simulink model "six_phase_half_wave_rectifier"  (R2022a)
settings: Solver=VariableStepAuto  StartTime=0.0  StopTime=0.04  FixedStep=1e-8  RelTol=1e-3
libraries: spsVoltageMeasurementLib x8, spsDetailedThyristorLib x6, spsACVoltageSourceLib x6, spsSeriesRLCBranchLib x1, spsCurrentMeasurementLib x1, spsGroundLib x1, spspowerguiLib x1
settings Model: Creator=alireza  LastModifiedBy=P.O.M.G
settings SolverCC: AlgebraicLoopSolver=TrustRegion
settings DataIOCC: ReturnWorkspaceOutputs=off
settings OptimizationCC: LifeSpan=inf
settings DebuggingCC: UnconnectedInputMsg=warning  UnconnectedOutputMsg=warning  UnconnectedLineMsg=warning  SFExecutionAtInitializationDiag=none  SFMachineParentedDataDiag=warning  ArithmeticOperatorsInVariantConditions=warning
settings SFSimCC: CustomCodeUndefinedFunction=UseInterfaceOnly
settings CodeAppCC: StateflowObjectComments=on

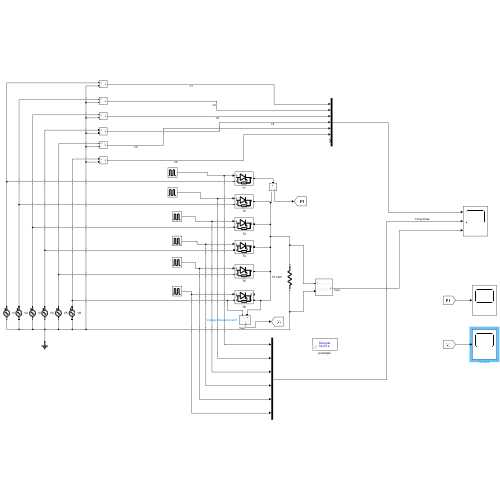
[thumbnail: Simulink's stored preview of the top-level diagram]
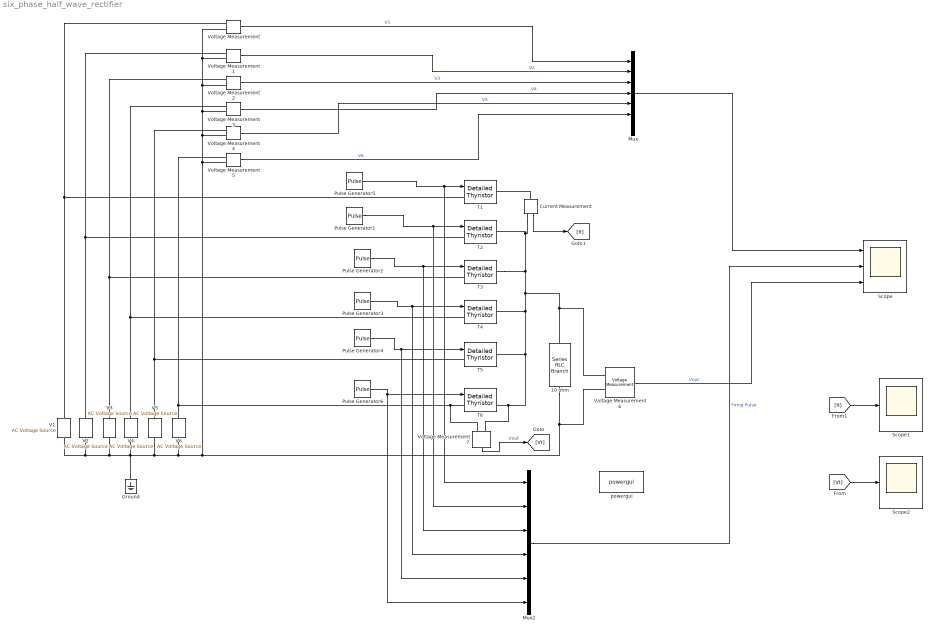
== system six_phase_half_wave_rectifier ==
  10 ohm : spsSeriesRLCBranchLib/Series RLC Branch  LConnTagsString=__new0  RConnTagsString=__new0  BranchType=R  Resistance=10  Inductance=1e-3  SetiL0=off  InitialCurrent=0  Capacitance=1e-6  Setx0=off  InitialVoltage=0  Measurements=None
  Current Measurement : spsCurrentMeasurementLib/Current Measurement  PhasorSimulation=off  OutputType=Complex  PSBequivalent=0
  Ground : spsGroundLib/Ground  LConnTagsString=a
  Mux : Mux  Inputs=7
  Mux2 : Mux  Inputs=6
  Pulse Generator1 : DiscretePulseGenerator  PulseType=Time based  Period=0.02  PulseWidth=5  PhaseDelay=0.02
  Pulse Generator2 : DiscretePulseGenerator  PulseType=Time based  Period=0.02  PulseWidth=5  PhaseDelay=0.01667
  Pulse Generator3 : DiscretePulseGenerator  PulseType=Time based  Period=0.02  PulseWidth=5  PhaseDelay=0.01333
  Pulse Generator4 : DiscretePulseGenerator  PulseType=Time based  Period=0.02  PulseWidth=5  PhaseDelay=0.01
  Pulse Generator5 : DiscretePulseGenerator  PulseType=Time based  Period=0.02  PulseWidth=5  PhaseDelay=0.00333
  Pulse Generator6 : DiscretePulseGenerator  PulseType=Time based  Period=0.02  PulseWidth=5  PhaseDelay=0.00667
  Scope : Scope  NumInputPorts=3
  Scope1 : Scope
  Scope2 : Scope
  T{1..5} (5 alike) : spsDetailedThyristorLib/Detailed Thyristor  Ron=0.001  Lon=1e-3  Vf=0.8  IL=0.1  Tq=100e-6  IC=0  Rs=500  Cs=250e-9  Measurements=off
      settings: SourceProductBaseCode=PS
  T6 : spsDetailedThyristorLib/Detailed Thyristor  Ron=0.001  Lon=1e-3  Vf=0.8  IL=0.1  Tq=100e-6  IC=0  Rs=500  Cs=250e-9  Measurements=on
      settings: SourceProductBaseCode=PS
  V1 : spsACVoltageSourceLib/AC Voltage Source  Amplitude=308  Phase=0  Frequency=50  SampleTime=0  Measurements=None  BusType=swing  Pref=10e3  Qref=0  Qmin=-inf  Qmax=+inf
  V2 : spsACVoltageSourceLib/AC Voltage Source  Amplitude=308  Phase=300  Frequency=50  SampleTime=0  Measurements=None  BusType=swing  Pref=10e3  Qref=0  Qmin=-inf  Qmax=+inf
  V3 : spsACVoltageSourceLib/AC Voltage Source  Amplitude=308  Phase=240  Frequency=50  SampleTime=0  Measurements=None  BusType=swing  Pref=10e3  Qref=0  Qmin=-inf  Qmax=+inf
  V4 : spsACVoltageSourceLib/AC Voltage Source  Amplitude=308  Phase=180  Frequency=50  SampleTime=0  Measurements=None  BusType=swing  Pref=10e3  Qref=0  Qmin=-inf  Qmax=+inf
  V5 : spsACVoltageSourceLib/AC Voltage Source  Amplitude=308  Phase=120  Frequency=50  SampleTime=0  Measurements=None  BusType=swing  Pref=10e3  Qref=0  Qmin=-inf  Qmax=+inf
  V6 : spsACVoltageSourceLib/AC Voltage Source  Amplitude=308  Phase=60  Frequency=50  SampleTime=0  Measurements=None  BusType=swing  Pref=10e3  Qref=0  Qmin=-inf  Qmax=+inf
  Voltage Measurement{,1..7} (8 alike) : spsVoltageMeasurementLib/Voltage Measurement  PhasorSimulation=off  OutputType=Complex  PSBequivalent=0
  powergui : spspowerguiLib/powergui  Priority=1  SimulationMode=Discrete  SampleTime=50e-6  frequency=60  Iterations=50  frequencyindice=50  Pbase=100e6  ErrMax=1e-4  UnitsV=kV  UnitsW=MW  buscounter=0  FunctionMessages=off  echomessages=off  EnableUseOfTLC=off  CurrentSourceSwitches=off  DisableSnubberDevices=off  DisableRonSwitches=off  DisableVfSwitches=off  DisplayEquations=off  AutomaticDiscreteSolvers=off  SolverType=Tustin/Backward Euler (TBE)  Interpol=off  ExternalGateDelay=off  methode=off  Ts=100  x0status=blocks  SPID=off  SwTol=0  HookPort=off  NonlinearTolerance=1e-4  nMaxIteration=100  ContinueOnMaxIteration=off  RestoreLinks=warning  ResistiveCurrentMeasurement=off  Frange=[0:2:500]  Ylog=off  Xlog=on  ShowGrid=off  save=off  variable=ZData  structure=0  ZoomFFT=off  StartTime=0.0  cycles=1  DisplayStyle=1  fundamental=60  FreqAxis=off  MaxFrequency=1000  frequencyindicesteady=1  RmsSteady=1  display=off
  wires:
  Voltage Measurement/1 -> Mux/1  "V1"
  Voltage Measurement1/1 -> Mux/2  "V2"
  Voltage Measurement2/1 -> Mux/3  "V3"
  Voltage Measurement3/1 -> Mux/4  "V4"
  Voltage Measurement4/1 -> Mux/5  "V5"
  Voltage Measurement5/1 -> Mux/6  "V6"
  Pulse Generator1/1 -> Mux2/2, T2/1
  Pulse Generator2/1 -> Mux2/3, T3/1
  Pulse Generator4/1 -> Mux2/5, T5/1
  Mux/1 -> Scope/1
  Pulse Generator5/1 -> Mux2/1, T1/1
  Pulse Generator6/1 -> Mux2/6, T6/1
  Mux2/1 -> Scope/2  "Firing Pulse"
  Pulse Generator3/1 -> Mux2/4, T4/1
  Voltage Measurement7/1 -> [Vt]  "Vout"
  Current Measurement/1 -> [It]
  [It] -> Scope1/1
  [Vt] -> Scope2/1
  Voltage Measurement6/1 -> Scope/3  "Vout"
  connections:
  Voltage Measurement/LConn2 -- Voltage Measurement1/LConn2 -- Voltage Measurement2/LConn2 -- Voltage Measurement3/LConn2 -- Voltage Measurement4/LConn2 -- Voltage Measurement6/LConn2 -- 10 ohm/RConn1 -- V5/LConn1 -- V1/LConn1 -- V2/LConn1 -- V3/LConn1 -- V4/LConn1 -- Ground/LConn1 -- V6/LConn1 -- Voltage Measurement5/LConn2
  Voltage Measurement/LConn1 -- V1/RConn1 -- T1/LConn1
  Voltage Measurement1/LConn1 -- T2/LConn1 -- V2/RConn1
  Voltage Measurement2/LConn1 -- T3/LConn1 -- V3/RConn1
  Voltage Measurement3/LConn1 -- T4/LConn1 -- V4/RConn1
  Voltage Measurement4/LConn1 -- T5/LConn1 -- V5/RConn1
  Voltage Measurement5/LConn1 -- T6/LConn1 -- Voltage Measurement7/LConn2 -- V6/RConn1
  T3/RConn1 -- Voltage Measurement6/LConn1 -- 10 ohm/LConn1 -- Voltage Measurement7/LConn1 -- T6/RConn1 -- T5/RConn1 -- T4/RConn1 -- Current Measurement/RConn1 -- T2/RConn1
  Current Measurement/LConn1 -- T1/RConn1
